simulink model "F16_2003hiModelAutopilotSim"  (R2013a)
settings: Solver=ode3  StartTime=0.0  StopTime=40  FixedStep=0.01  RelTol=1e-5
InitFcn:
  | F16_2003hiModelAutopilot
values from neighbouring files (symbols this model uses):
  A = [0	0	0	0	0	0	1	0	0	0	0	0	0	0	0	0	0	0 ... (first row only)    [F16NolinearModelRemoveWindControlData_low.m]    (also in F16_2003hiModelAutopilot.m = [0	0	0	0	-2.55E-09	0	1	0	0	0	0	0	0	0	0	0	0	0; F16_2003hiModelAutopilot1.m = [0	0	0	0	-2.55E-09	0	1	0	0	0	0	0	0	0	0	0	0	0; F16_2003hiModelAutopilot1_steadySys.m = [0	0	0	0	-2.55E-09	0	1	0	0	0	0	0	0	0	0	0	0	0; LQR_Calc2.m = [A1,zeros(8,2);-C_v_theta,zeros(2,2)])
  A_la = A([2,4,6,9,10,12,15,16],[2,4,6,9,10,12,15,16])    [F16NolinearModelRemoveWindControlData_low.m]    (also in F16_2003hiModelAutopilot.m; F16_2003hiModelAutopilot1.m; F16_2003hiModelAutopilot1_steadySys.m = A([4,6,9,10,12,15,16],[4,6,9,10,12,15,16]); LQR_Calc2_F16YingHu_lonAndLa.m = A_full(8:12,8:12))
  A_lon = A([1,3,5,7,8,11,13,14],[1,3,5,7,8,11,13,14])    [F16NolinearModelRemoveWindControlData_low.m]    (also in F16_2003hiModelAutopilot.m; F16_2003hiModelAutopilot1.m; F16_2003hiModelAutopilot1_steadySys.m = A([5,7,8,11,13,14],[5,7,8,11,13,14]); LQR_Calc2_F16YingHu_lonAndLa.m = A_full(1:7,1:7))
  B = [0	0	0	0 ... (first row only)    [F16NolinearModelRemoveWindControlData_low.m]    (also in F16_2003hiModelAutopilot.m; F16_2003hiModelAutopilot1.m; F16_2003hiModelAutopilot1_steadySys.m; LQR_Calc2.m = [B1;zeros(2,2)])
  B_la = B([2,4,6,9,10,12,15,16],3:4)    [F16NolinearModelRemoveWindControlData_low.m]    (also in F16_2003hiModelAutopilot.m; F16_2003hiModelAutopilot1.m; F16_2003hiModelAutopilot1_steadySys.m = B([4,6,9,10,12,15,16],3:4); LQR_Calc2_F16YingHu_lonAndLa.m = B_full(8:12,3:4))
  B_lon = B([1,3,5,7,8,11,13,14],1:2)    [F16NolinearModelRemoveWindControlData_low.m]    (also in F16_2003hiModelAutopilot.m; F16_2003hiModelAutopilot1.m; F16_2003hiModelAutopilot1_steadySys.m = B([5,7,8,11,13,14],1:2); LQR_Calc2_F16YingHu_lonAndLa.m = B_full(1:7,1:2))
  C = [1,zeros(1,17) ... (first row only)    [F16NolinearModelRemoveWindControlData_low.m]    (also in F16_2003hiModelAutopilot.m; F16_2003hiModelAutopilot1.m; F16_2003hiModelAutopilot1_steadySys.m; LQR_Calc2.m = [-C_v_theta,zeros(2,2)])
  C_la_yd = [1 zeros(1,7)]    [F16NolinearModelRemoveWindControlData_low.m]    (also in F16_2003hiModelAutopilot.m; F16_2003hiModelAutopilot1.m)
  C_lon_xd_h = [1 zeros(1,7) ... (first row only)    [F16NolinearModelRemoveWindControlData_low.m]    (also in F16_2003hiModelAutopilot.m; F16_2003hiModelAutopilot1.m)
  Ki = zeros(4,3)    [F16NolinearModelRemoveWindControlData_low.m]    (also in F16_2003hiModelAutopilot.m; F16_2003hiModelAutopilot1.m; LQR_Calc2.m = -k(:,9:10); LQR_Calc2LowPrecision.m = -k(:,9:10))
  Ki_la = -k_la(:,9)    [F16NolinearModelRemoveWindControlData_low.m]    (also in F16_2003hiModelAutopilot.m; F16_2003hiModelAutopilot1.m; LQR_Calc2_F16YingHu_lonAndLa.m = -k_la(:,6))
  Ki_lon = -k_lon(:,9:10)    [F16NolinearModelRemoveWindControlData_low.m]    (also in F16_2003hiModelAutopilot.m; F16_2003hiModelAutopilot1.m; LQR_Calc2_F16YingHu_lonAndLa.m = -k_lon(:,8:9))
  Kp = zeros(4,18)    [F16NolinearModelRemoveWindControlData_low.m]    (also in F16_2003hiModelAutopilot.m; F16_2003hiModelAutopilot1.m; F16_2003hiModelAutopilot1_steadySys.m; LQR_Calc2.m = k(:,1:8))
  Kp_la = k_la(:,1:8)    [F16NolinearModelRemoveWindControlData_low.m]    (also in F16_2003hiModelAutopilot.m; F16_2003hiModelAutopilot1.m; F16_2003hiModelAutopilot1_steadySys.m = k_la; LQR_Calc2_F16YingHu_lonAndLa.m = k_la(:,1:5))
  Kp_lon = k_lon(:,1:8)    [F16NolinearModelRemoveWindControlData_low.m]    (also in F16_2003hiModelAutopilot.m; F16_2003hiModelAutopilot1.m; F16_2003hiModelAutopilot1_steadySys.m = k_lon; LQR_Calc2_F16YingHu_lonAndLa.m = k_lon(:,1:7))
settings Model: Creator=Dai  LastModifiedBy=Dai

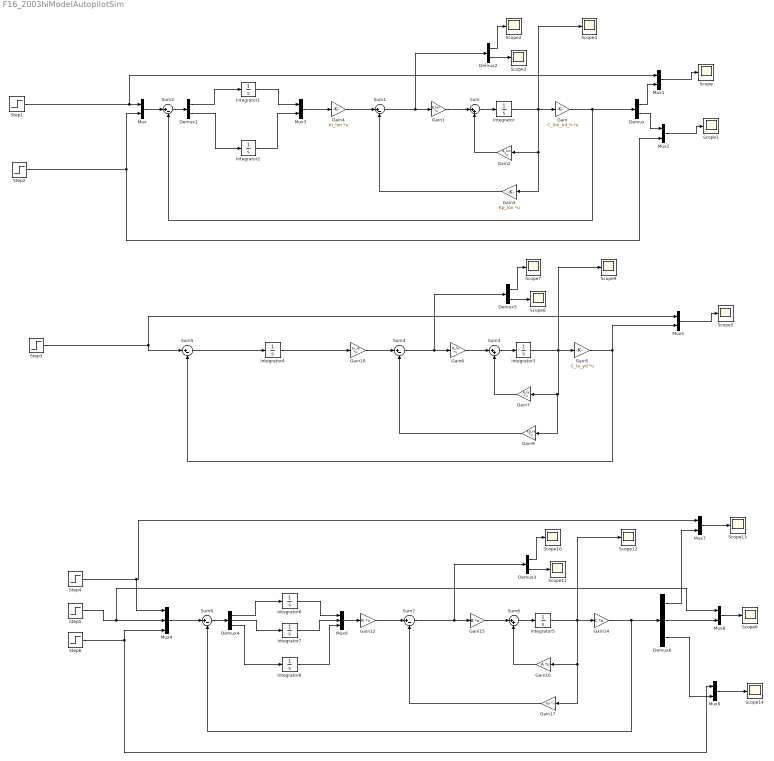
== system F16_2003hiModelAutopilotSim ==
  Demux{,1..3,5} (5 alike) : Demux  Outputs=2
  Demux4 : Demux  Outputs=3
  Demux6 : Demux  Outputs=3
  Gain : Gain  Gain=C_lon_xd_h  Multiplication=Matrix(K*u) (u vector)
  Gain1 : Gain  Gain=B_lon  Multiplication=Matrix(K*u) (u vector)
  Gain10 : Gain  Gain=Ki_la  Multiplication=Matrix(K*u) (u vector)
  Gain12 : Gain  Gain=Ki  Multiplication=Matrix(K*u) (u vector)
  Gain14 : Gain  Gain=C  Multiplication=Matrix(K*u) (u vector)
  Gain15 : Gain  Gain=B  Multiplication=Matrix(K*u) (u vector)
  Gain16 : Gain  Gain=A  Multiplication=Matrix(K*u) (u vector)
  Gain17 : Gain  Gain=Kp  Multiplication=Matrix(K*u) (u vector)
  Gain2 : Gain  Gain=A_lon  Multiplication=Matrix(K*u) (u vector)
  Gain3 : Gain  Gain=Kp_lon  Multiplication=Matrix(K*u) (u vector)
  Gain4 : Gain  Gain=Ki_lon  Multiplication=Matrix(K*u) (u vector)
  Gain5 : Gain  Gain=C_la_yd  Multiplication=Matrix(K*u) (u vector)
  Gain6 : Gain  Gain=B_la  Multiplication=Matrix(K*u) (u vector)
  Gain7 : Gain  Gain=A_la  Multiplication=Matrix(K*u) (u vector)
  Gain9 : Gain  Gain=Kp_la  Multiplication=Matrix(K*u) (u vector)
  Integrator{,1..8} (9 alike) : Integrator
  Mux{,1..3,5,7..9} (8 alike) : Mux  Inputs=2
  Mux4 : Mux  Inputs=3
  Mux6 : Mux  Inputs=3
  Scope{,1..14} (15 alike) : Scope
      Scope10 settings: SaveName=ScopeData6
      Scope11 settings: SaveName=ScopeData10
      Scope12 settings: SaveName=ScopeData11
      Scope13 settings: TimeRange=10  YMin=-1  YMax=1  SaveName=ScopeData13
      Scope14 settings: SaveName=ScopeData14
      Scope2 settings: SaveName=ScopeData2
      Scope3 settings: SaveName=ScopeData3
      Scope4 settings: SaveName=ScopeData4
      Scope5 settings: SaveName=ScopeData5
      Scope6 settings: SaveName=ScopeData12
      Scope7 settings: SaveName=ScopeData7
      Scope8 settings: SaveName=ScopeData8
      Scope9 settings: SaveName=ScopeData9
  Step1 : Step  Time=10  After=10  SampleTime=0
  Step2 : Step  After=2  SampleTime=0
  Step3 : Step  Time=0  SampleTime=0
  Step4 : Step  Time=20  After=10  SampleTime=0
  Step5 : Step  Time=2  After=2  SampleTime=0
  Step6 : Step  Time=2  After=0  SampleTime=0
  Sum : Sum  Inputs=|++
  Sum{1..2,4..5,7..8} (6 alike) : Sum  Inputs=|+-
  Sum3 : Sum  Inputs=|++
  Sum6 : Sum  Inputs=|++
  wires:
  Integrator/1 -> Scope4/1, Gain3/1, Gain2/1, Gain/1
  Gain1/1 -> Sum/1
  Sum/1 -> Integrator/1
  Gain2/1 -> Sum/2
  Sum1/1 -> Demux2/1, Gain1/1
  Gain4/1 -> Sum1/1
  Gain/1 -> Demux/1, Sum2/2
  Mux/1 -> Sum2/1
  Step1/1 -> Mux1/1, Mux/1
  Demux/1 -> Mux1/2
  Mux1/1 -> Scope/1
  Step2/1 -> Mux/2, Mux2/2
  Mux2/1 -> Scope1/1
  Demux/2 -> Mux2/1
  Gain3/1 -> Sum1/2
  Sum2/1 -> Demux1/1
  Mux3/1 -> Gain4/1
  Demux1/1 -> Integrator1/1
  Integrator1/1 -> Mux3/1
  Demux1/2 -> Integrator2/1
  Integrator2/1 -> Mux3/2
  Demux2/1 -> Scope2/1
  Demux2/2 -> Scope3/1
  Integrator3/1 -> Scope9/1, Gain9/1, Gain7/1, Gain5/1
  Gain6/1 -> Sum3/1
  Sum3/1 -> Integrator3/1
  Gain7/1 -> Sum3/2
  Sum4/1 -> Demux5/1, Gain6/1
  Gain10/1 -> Sum4/1
  Gain5/1 -> Mux5/2, Sum5/2
  Step3/1 -> Sum5/1, Mux5/1
  Mux5/1 -> Scope5/1
  Gain9/1 -> Sum4/2
  Sum5/1 -> Integrator4/1
  Demux5/1 -> Scope7/1
  Demux5/2 -> Scope8/1
  Integrator4/1 -> Gain10/1
  Integrator5/1 -> Scope12/1, Gain17/1, Gain16/1, Gain14/1
  Gain15/1 -> Sum6/1
  Sum6/1 -> Integrator5/1
  Gain16/1 -> Sum6/2
  Sum7/1 -> Demux3/1, Gain15/1
  Gain14/1 -> Sum8/2, Demux6/1
  Gain17/1 -> Sum7/2
  Demux3/1 -> Scope10/1
  Demux3/2 -> Scope11/1
  Sum8/1 -> Demux4/1
  Mux6/1 -> Gain12/1
  Demux4/1 -> Integrator6/1
  Integrator6/1 -> Mux6/1
  Demux4/2 -> Integrator7/1
  Integrator7/1 -> Mux6/2
  Demux4/3 -> Integrator8/1
  Integrator8/1 -> Mux6/3
  Step4/1 -> Mux4/1, Mux7/1
  Step5/1 -> Mux8/1, Mux4/2
  Step6/1 -> Mux4/3, Mux9/1
  Demux6/1 -> Mux7/2
  Demux6/2 -> Mux8/2
  Mux8/1 -> Scope6/1
  Demux6/3 -> Mux9/2
  Mux7/1 -> Scope13/1
  Mux9/1 -> Scope14/1
  Gain12/1 -> Sum7/1
  Mux4/1 -> Sum8/1
